simulink model "ballBeamSimulink"  (R2025b)
settings: Solver=ode2  StartTime=0.0  StopTime=100  FixedStep=1e-3  RelTol=1e-3
undefined symbols (not defined in the file): Den, Kd, Ki, Kp, Num
settings Model: Creator=omari  LastModifiedBy=omari

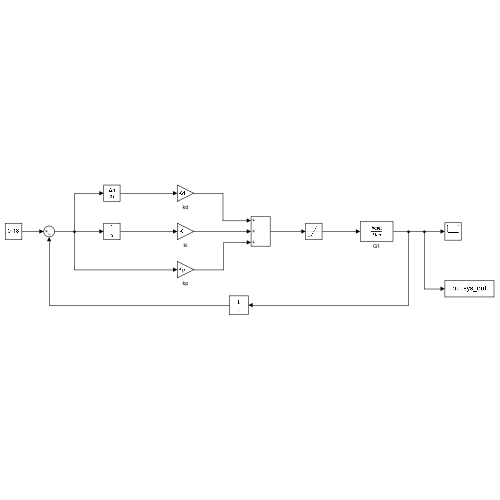
[thumbnail: Simulink's stored preview of the top-level diagram]
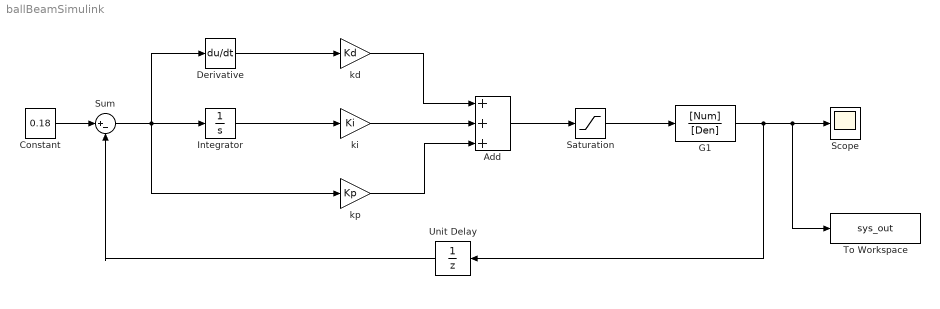
== system ballBeamSimulink ==
  Add : Sum  Inputs=+++
  Constant : Constant  Value=0.18
  Derivative : Derivative
  G1 : TransferFcn  Numerator=[Num]  Denominator=[Den]
  Integrator : Integrator
  Saturation : Saturate  UpperLimit=0.698132  LowerLimit=-0.698132
  Scope : Scope
      settings: ActiveDisplayYMinimum=-0.022500134156945649  ActiveDisplayYMaximum=0.20250120741251088
  Sum : Sum  Inputs=|+-
  To Workspace : ToWorkspace  VariableName=sys_out  SaveFormat=Timeseries  SampleTime=-1
  Unit Delay : UnitDelay  SampleTime=-1  HasFrameUpgradeWarning=on
  kd : Gain  Gain=Kd
  ki : Gain  Gain=Ki
  kp : Gain  Gain=Kp
  wires:
  kp/1 -> Add/3
  Add/1 -> Saturation/1
  Sum/1 -> Derivative/1, Integrator/1, kp/1
  G1/1 -> To Workspace/1, Scope/1, Unit Delay/1
  Constant/1 -> Sum/1
  Unit Delay/1 -> Sum/2
  Integrator/1 -> ki/1
  Derivative/1 -> kd/1
  kd/1 -> Add/1
  ki/1 -> Add/2
  Saturation/1 -> G1/1
